simulink model "AmpelkreuzungV4_8"  (R2024b)
settings: Solver=FixedStepAuto  StartTime=0.0  StopTime=1000  FixedStep=1  RelTol=1e-3
model workspace (MATLAB code in the model file):
  | function [autos_l1, autos_rg1, autos_2l, autos_2rg, autos_3l, autos_3rg, autos_4, fehler] = generateCars(Auslastung)
  |     if (auslastung == 1)
  |         autos_l1 = round(randn());
  |         autos_rg1 = round(randn());
  |         autos_2l = round(randn());
  |         autos_2rg = round(randn());
  |         autos_3l = round(randn());
  |         autos_3rg = round(randn());
  |         autos_4 = round(randn());
  |     else
  |         fehler = 1;
  |     end
  | 
  |     if (auslastung == 2)
  |         autos_l1 = round(randn());
  |         autos_rg1 = round(4 + 2 * randn());
  |         autos_2l = round(1 + randn());
  |         autos_2rg = round(4 + 2 * randn());
  |         autos_3l = round(randn());
  |         autos_3rg = round(2 + randn());
  |         autos_4 = round(1 + randn());
  |     else
  |         fehler = 1;
  |     end
  | 
  |     if (auslastung == 3)
  |         autos_l1 = round(1.5 + randn());
  |         autos_rg1 = round(7 + 2 * randn());
  |         autos_2l = round(2 + randn());
  |         autos_2rg = round(7 + 2 * randn());
  |         autos_3l = round(2 * randn());
  |         autos_3rg = round(3 + randn());
  |         autos_4 = round(2 + randn());
  |     else
  |         fehler = 1;
  |     end
  | 
  |     if (auslastung == 4)
  |         autos_l1 = round(2.5 + randn());
  |         autos_rg1 = round(13 + 3 * randn());
  |         autos_2l = round(5 + randn());
  |         autos_2rg = round(13 + 3 * randn());
  |         autos_3l = round(2 + randn());
  |         autos_3rg = round(2 + randn());
  |         autos_4 = round(5 + randn());
  |     else
  |         fehler = 1;
  |     end
  | end
(part 1 of 2)
settings Model: PacingRate=1000  Creator=richa  LastModifiedBy=richa

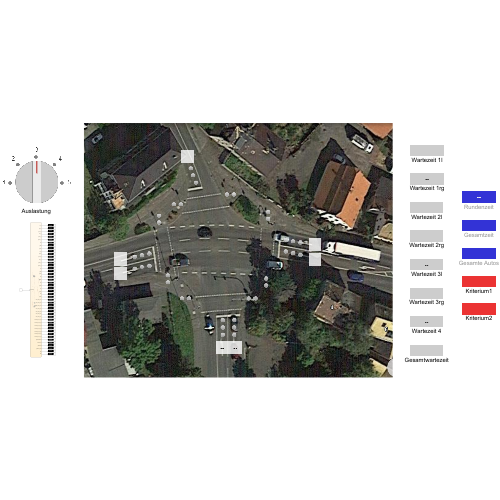
[thumbnail: Simulink's stored preview of the top-level diagram]
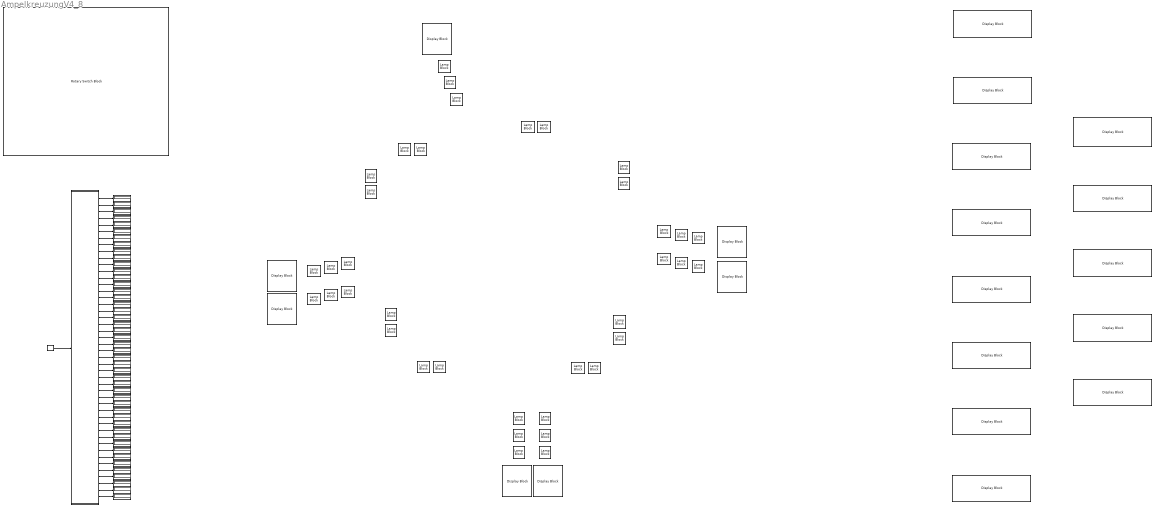
== system AmpelkreuzungV4_8 ==
  Auslastung : RotarySwitchBlock  LabelPosition=Hide
      settings: Values={{'1', '2', '3', '4', '5'}, [1 2 3 4 5]}
  Chart : Stateflow chart  TreatAsAtomicUnit=on
  Constant : Constant  Value=3
  Display{,1..26,28..33,38,41..52} (46 alike) : Display
  Display{27,34..37,39..40} (7 alike) : DisplayBlock  LabelPosition=Hide  Transparency=1  Layout=Fill available space
  Gesamte Autos : DisplayBlock  LabelPosition=Hide  Transparency=1
  Gesamtwartezeit : DisplayBlock  LabelPosition=Hide  Transparency=1
  Gesamtzeit : DisplayBlock  LabelPosition=Hide  Transparency=1
  Kriterium1 : DisplayBlock  LabelPosition=Hide  Transparency=1
  Kriterium2 : DisplayBlock  LabelPosition=Hide  Transparency=1
  Lamp{,1..36} (37 alike) : LampBlock  LabelPosition=Hide
  Rundenzeit : DisplayBlock  LabelPosition=Hide  Transparency=1
  Wartezeit 1l : DisplayBlock  LabelPosition=Hide  Transparency=1
  Wartezeit 1rg : DisplayBlock  LabelPosition=Hide  Transparency=1
  Wartezeit 2l : DisplayBlock  LabelPosition=Hide  Transparency=1
  Wartezeit 2rg : DisplayBlock  LabelPosition=Hide  Transparency=1
  Wartezeit 3l : DisplayBlock  LabelPosition=Hide  Transparency=1
  Wartezeit 3rg : DisplayBlock  LabelPosition=Hide  Transparency=1
  Wartezeit 4 : DisplayBlock  LabelPosition=Hide  Transparency=1
  wires:
  Chart/26(gruen8) -> Display25/1
  Chart/10(rot3_l) -> Display9/1
  Chart/24(gruen7) -> Display23/1
  Chart/4(rot1_rg) -> Display3/1
  Chart/11(gelb3_l) -> Display10/1
  Chart/5(gelb1_rg) -> Display4/1
  Chart/9(gruen2) -> Display8/1
  Chart/13(rot3_rg) -> Display12/1
  Chart/25(rot8) -> Display24/1
  Chart/20(gruen5) -> Display19/1
  Chart/12(gruen3_l) -> Display11/1
  Constant/1 -> Chart/1(auslastung)
  Chart/2(gelb1_l) -> Display1/1
  Chart/21(rot6) -> Display20/1
  Chart/8(gelb2) -> Display7/1
  Chart/6(gruen1_rg) -> Display5/1
  Chart/15(gruen3_rg) -> Display14/1
  Chart/43(gesamtZeit) -> Display42/1
  Chart/42(timeCounter) -> Display38/1
  Chart/16(rot4) -> Display15/1
  Chart/1(rot1_l) -> Display/1
  Chart/14(gelb3_rg) -> Display13/1
  Chart/23(rot7) -> Display22/1
  Chart/3(gruen1_l) -> Display2/1
  Chart/7(rot2) -> Display6/1
  Chart/19(rot5) -> Display18/1
  Chart/22(gruen6) -> Display21/1
  Chart/17(gelb4) -> Display16/1
  Chart/18(gruen4) -> Display17/1
  Chart/28(autos_auf_spur2) -> Display45/1
  Chart/27(autos_auf_spur1) -> Display51/1
  Chart/29(autos_auf_spur3) -> Display46/1
  Chart/30(autos_auf_spur4) -> Display47/1
  Chart/31(autos_auf_spur5) -> Display48/1
  Chart/32(autos_auf_spur6) -> Display49/1
  Chart/33(autos_auf_spur7) -> Display50/1
  Chart/35(wartezeit_spur2_ges) -> Display28/1
  Chart/34(wartezeit_spur1_ges) -> Display26/1
  Chart/44(gesamte_autos) -> Display29/1
  Chart/36(wartezeit_spur3_ges) -> Display44/1
  Chart/39(wartezeit_spur6_ges) -> Display32/1
  Chart/37(wartezeit_spur4_ges) -> Display30/1
  Chart/38(wartezeit_spur5_ges) -> Display31/1
  Chart/40(wartezeit_spur7_ges) -> Display33/1
  Chart/41(gesamtwartezeit) -> Display41/1
  Chart/45(krit1) -> Display43/1
  Chart/46(krit2) -> Display52/1
